simulink model "System"  (R2023b)
settings: Solver=VariableStepAuto  StartTime=0.0  StopTime=10.0  RelTol=1e-3
settings Model: Creator=visha  LastModifiedBy=visha
settings OptimizationCC: DefaultParameterBehavior=Inlined

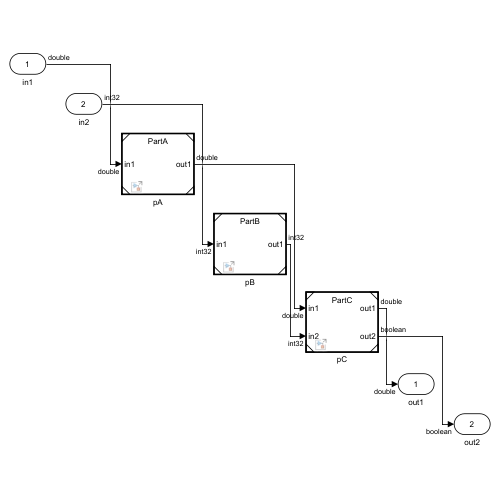
[thumbnail: Simulink's stored preview of the top-level diagram]
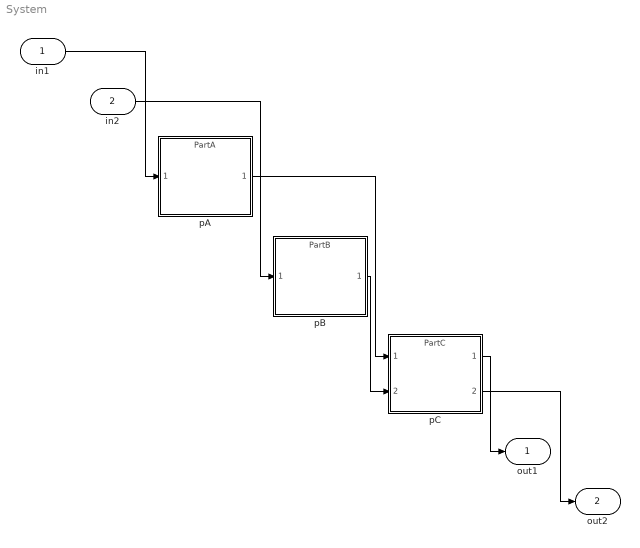
== system System ==
  in1 : Inport  OutDataTypeStr=double
  in2 : Inport  Port=2  OutDataTypeStr=int32
  pA : ModelReference  ModelNameDialog=PartA  SimulationMode=Normal  ModelReferenceVersion=1.1
  pB : ModelReference  ModelNameDialog=PartB  SimulationMode=Normal  ModelReferenceVersion=1.1
  pC : ModelReference  ModelNameDialog=PartC  SimulationMode=Normal  ModelReferenceVersion=1.1
  out1 : Outport  OutDataTypeStr=double
  out2 : Outport  Port=2  OutDataTypeStr=boolean
  wires:
  in1/1 -> pA/1
  in2/1 -> pB/1
  pA/1 -> pC/1
  pB/1 -> pC/2
  pC/1 -> out1/1
  pC/2 -> out2/1
